simulink model "Testing_Model"  (R2020b)
settings: Solver=VariableStepAuto  StartTime=0.0  StopTime=inf  RelTol=1e-3
libraries: instrumentlib x2, dspstat3 x1, dspindex x1, realtime_pacer_lib x1, SignalEditorBlockLib x1
settings Model: Creator=errikos  LastModifiedBy=errikoslevis
settings DataIOCC: ReturnWorkspaceOutputs=off
settings DebuggingCC: ArithmeticOperatorsInVariantConditions=warning
settings SFSimCC: CustomCodeUndefinedFunction=UseInterfaceOnly

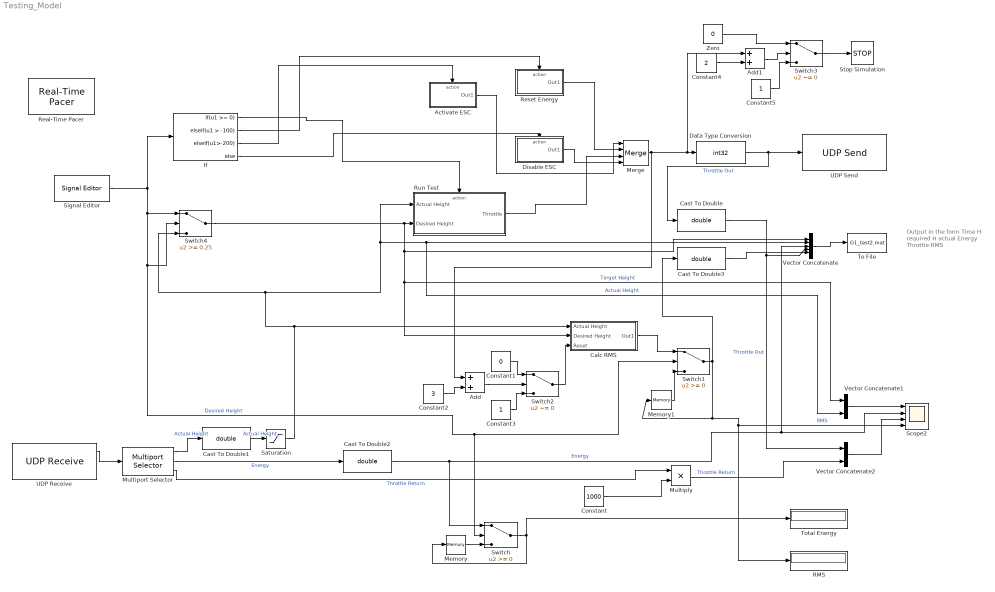
== system Testing_Model ==
  note: Output in the form
      | Time
      | H required
      | H actual
      | Energy
      | Throttle
      | RMS
  Activate ESC : Subsystem  TreatAsAtomicUnit=on
  Add : Sum
  Add1 : Sum
  Calc RMS : Subsystem
  Cast To Double{,1..3} (4 alike) : DataTypeConversion  OutDataTypeStr=double
  Constant : Constant  Value=1000
  Constant1 : Constant  Value=0
  Constant2 : Constant  Value=3
  Constant3 : Constant
  Constant4 : Constant  Value=2
  Constant5 : Constant
  Data Type Conversion : DataTypeConversion  OutDataTypeStr=int32
  Disable ESC : Subsystem  TreatAsAtomicUnit=on
  If : If  IfExpression=u1 >= 0  ElseIfExpressions=u1 > -100 , u1>-200
  Memory : Memory
  Memory1 : Memory
  Merge : Merge  Inputs=4
  Multiply : Product
  Multiport Selector : dspindex/Multiport Selector  rowsOrCols=Columns  idxCellArray={ 1, 2,3}  idxErrMode=Clip and Warn
  RMS : Display
  Real-Time Pacer : realtime_pacer_lib/Real-Time Pacer  simTimePerRealTime=1
  Reset Energy : Subsystem  TreatAsAtomicUnit=on
  Run Test : Subsystem  TreatAsAtomicUnit=on
  Saturation : Saturate  UpperLimit=1.7  LowerLimit=0.1
  Scope2 : Scope  NumInputPorts=4
  Signal Editor : SignalEditorBlockLib/Signal Editor  FileName=/Users/errikoslevis/OneDrive - Imperial College London/Teaching/Duocopter Des Ex/2020-21/Scripts/Simulink/samplemission.mat  ActiveScenario=Scenario  ActiveSignal=Signal 1  IsBus=off  OutputBusObjectStr=Bus: BusObject  SampleTime=0.05  ZeroCross=off  OutputAfterFinalValue=Setting to zero  Unit=inherit  PreserveSignalName=on
  Stop Simulation : Stop
  Switch : Switch
  Switch1 : Switch
  Switch2 : Switch  Criteria=u2 ~= 0
  Switch3 : Switch  Criteria=u2 ~= 0  ZeroCross=off
  Switch4 : Switch  Threshold=0.25
  To File : ToFile  Filename=G1_test2.mat
  Total Energy : Display
  UDP Receive : instrumentlib/UDP Receive  Host=192.168.1.110  Port=4000  LocalPort=8888  EnablePortSharing=on  GetLatestData=on  DataSize="[1  3]"  DataType=single  ASCIIFormatting=%f%f  Terminator=LF  ByteOrder=LittleEndian  EnableBlockingMode=off  Timeout=10  SampleTime=0.005  LocalAddress=192.168.1.120
  UDP Send : instrumentlib/UDP Send  Host=192.168.1.110  Port=4000  LocalPort=-1  EnablePortSharing=on  ByteOrder=LittleEndian  OutputDatagramPacketSize=4  EnableBlockingMode=on  LocalAddress=192.168.1.120
  Vector Concatenate : Concatenate  NumInputs=5
  Vector Concatenate1 : Concatenate
  Vector Concatenate2 : Concatenate
  Zero : Constant  Value=0  OutDataTypeStr=Inherit: Inherit via back propagation
  wires:
  UDP Receive/1 -> Multiport Selector/1
  Multiport Selector/1 -> Cast To Double1/1  "Actual Height"
  Multiport Selector/2 -> Cast To Double2/1  "Energy"
  Run Test/1("Throttle ") -> Merge/3
  Data Type Conversion/1 -> Cast To Double/1, UDP Send/1  "Throttle Out"
  Multiport Selector/3 -> Multiply/1  "Throttle Return"
  Multiply/1 -> Vector Concatenate2/2  "Throttle Return"
  Constant/1 -> Multiply/2
  Signal Editor/1 -> Switch4/2, Switch1/2, Switch/2, Switch4/1, If/1  "Desired Height"
  Merge/1 -> Add/1, Add1/1, Data Type Conversion/1
  Vector Concatenate/1 -> To File/1
  If/1 -> Run Test/Action
  If/2 -> Reset Energy/Action
  If/3 -> Activate ESC/Action
  If/4 -> Disable ESC/Action
  Activate ESC/1(Out1) -> Merge/1
  Disable ESC/1(Out1) -> Merge/4
  Switch/1 -> Memory/1, Total Energy/1
  Cast To Double/1 -> Vector Concatenate2/1, Vector Concatenate/4  "Throttle Out"
  Saturation/1 -> Switch4/3, Run Test/1(Actual Height), Vector Concatenate1/2, Vector Concatenate/2, Calc RMS/1(Actual Height)  "Actual Height"
  Cast To Double2/1 -> Switch/1, Scope2/2, Vector Concatenate/3  "Energy"
  Cast To Double3/1 -> Vector Concatenate/5
  Memory/1 -> Switch/3
  Switch1/1 -> RMS/1, Scope2/4, Memory1/1, Cast To Double3/1  "RMS"
  Memory1/1 -> Switch1/3
  Calc RMS/1(Out1) -> Switch1/1
  Switch2/1 -> Calc RMS/3(Reset)
  Constant1/1 -> Switch2/1
  Constant2/1 -> Add/2
  Add/1 -> Switch2/2
  Constant3/1 -> Switch2/3
  Reset Energy/1(Out1) -> Merge/2
  Switch3/1 -> Stop Simulation/1
  Zero/1 -> Switch3/1
  Add1/1 -> Switch3/2
  Constant4/1 -> Add1/2
  Constant5/1 -> Switch3/3
  Vector Concatenate2/1 -> Scope2/3
  Vector Concatenate1/1 -> Scope2/1
  Switch4/1 -> Vector Concatenate/1, Vector Concatenate1/1, Calc RMS/2(Desired Height), Run Test/2(Desired Height)  "Target Height"
  Cast To Double1/1 -> Saturation/1  "Actual Height"

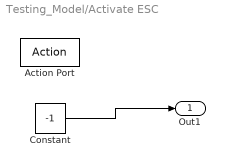
== system Testing_Model/Activate ESC ==
  Action Port : ActionPort  ActionPortLabel=elseif { }
  Constant : Constant  Value=-1  SampleTime=0.05
  Out1 : Outport  VectorParamsAs1DForOutWhenUnconnected=off
  wires:
  Constant/1 -> Out1/1

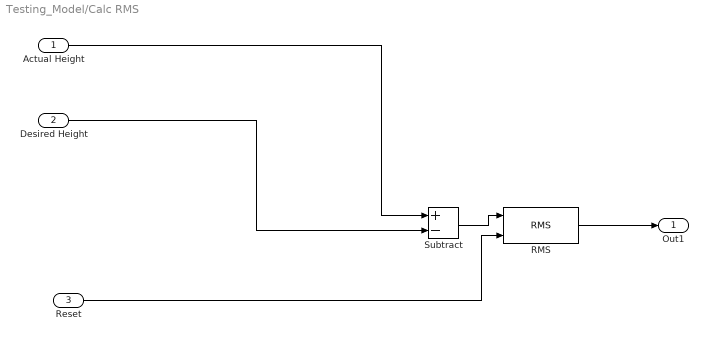
== system Testing_Model/Calc RMS ==
  Actual Height : Inport
  Desired Height : Inport  Port=2
  Reset : Inport  Port=3
  RMS : dspstat3/RMS  run=on  directionMode=Each column  dimension=1  reset_popup=Non-zero sample
  Subtract : Sum  Inputs=+-
  Out1 : Outport  VectorParamsAs1DForOutWhenUnconnected=off
  wires:
  Desired Height/1 -> Subtract/2
  Actual Height/1 -> Subtract/1
  RMS/1 -> Out1/1
  Subtract/1 -> RMS/1
  Reset/1 -> RMS/2

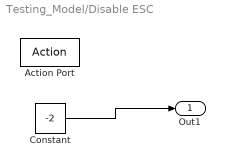
== system Testing_Model/Disable ESC ==
  Action Port : ActionPort  ActionPortLabel=else { }
  Constant : Constant  Value=-2  SampleTime=0.05
  Out1 : Outport  VectorParamsAs1DForOutWhenUnconnected=off
  wires:
  Constant/1 -> Out1/1

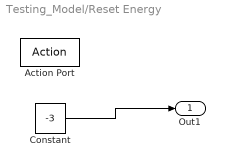
== system Testing_Model/Reset Energy ==
  Action Port : ActionPort  ActionPortLabel=elseif { }
  Constant : Constant  Value=-3  SampleTime=0.05
  Out1 : Outport  VectorParamsAs1DForOutWhenUnconnected=off
  wires:
  Constant/1 -> Out1/1

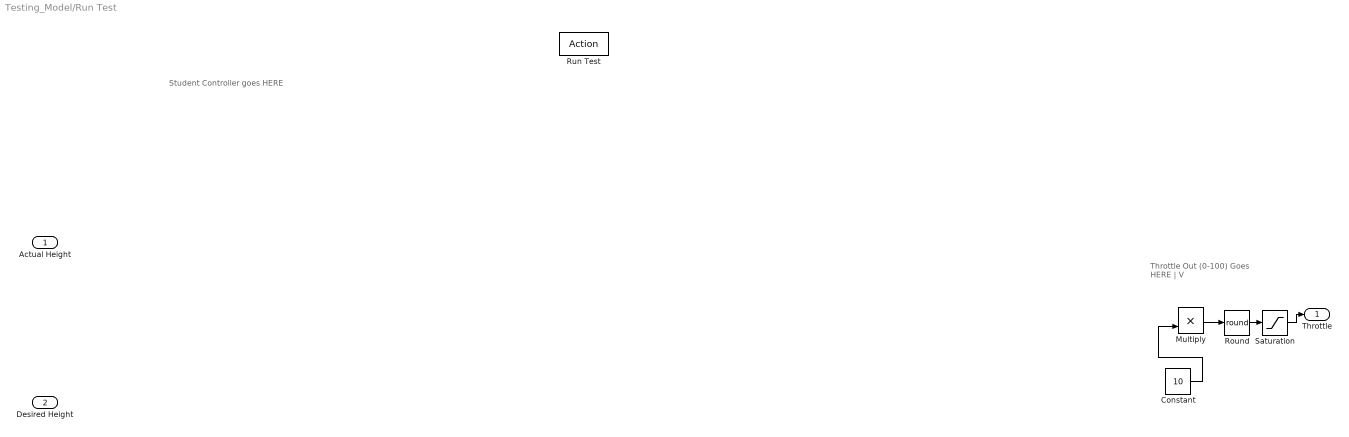
== system Testing_Model/Run Test ==
  note: Throttle Out (0-100)
      | Goes HERE
      |            |
      | 	   V
  note: Student Controller goes HERE
  Actual Height : Inport
  Desired Height : Inport  Port=2
  Run Test : ActionPort  ActionPortLabel=if { }
  Constant : Constant  Value=10
  Multiply : Product
  Round : Rounding  Operator=round
  Saturation : Saturate  UpperLimit=1000  LowerLimit=0
  "Throttle " : Outport  VectorParamsAs1DForOutWhenUnconnected=off
  wires:
  Saturation/1 -> "Throttle "/1
  Constant/1 -> Multiply/2
  Multiply/1 -> Round/1
  Round/1 -> Saturation/1
